simulink model "Hand_Made_PID"  (R2019a)
settings: Solver=VariableStepAuto  StartTime=0.0  StopTime=10.0  RelTol=1e-3
settings Model: Creator=hodam  LastModifiedBy=hodam

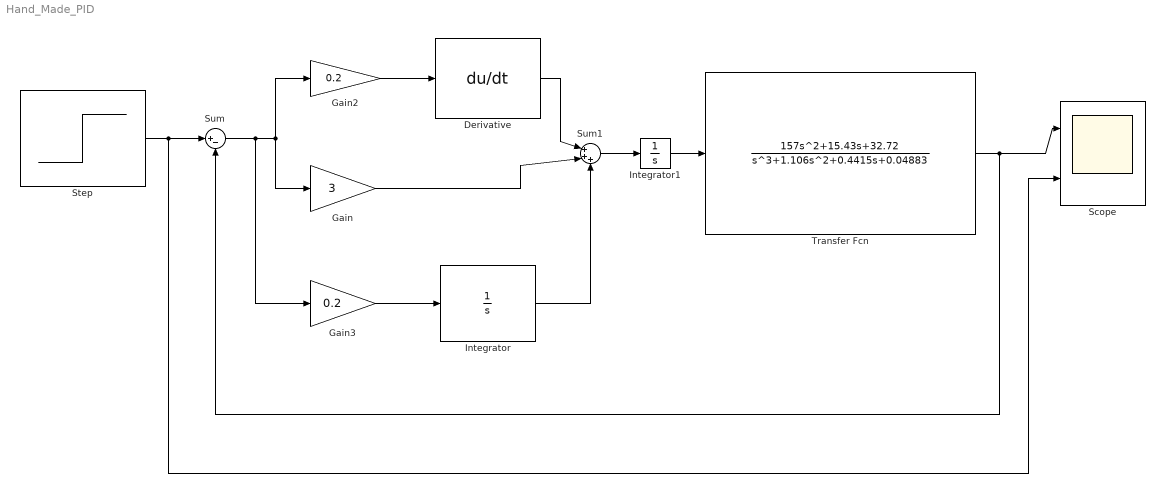
== system Hand_Made_PID ==
  Derivative : Derivative
  Gain : Gain  Gain=3
  Gain2 : Gain  Gain=0.2
  Gain3 : Gain  Gain=0.2
  Integrator : Integrator
  Integrator1 : Integrator
  Scope : Scope  NumInputPorts=2
  Step : Step  Time=0  After=60  SampleTime=0
  Sum : Sum  Inputs=|+-
  Sum1 : Sum  Inputs=|+++
  Transfer Fcn : TransferFcn  Numerator=[157 15.43 32.72]  Denominator=[1 1.106 0.4415 0.04883]
  wires:
  Derivative/1 -> Sum1/1
  Integrator/1 -> Sum1/3
  Gain/1 -> Sum1/2
  Gain3/1 -> Integrator/1
  Gain2/1 -> Derivative/1
  Sum/1 -> Gain3/1, Gain2/1, Gain/1
  Transfer Fcn/1 -> Sum/2, Scope/1
  Sum1/1 -> Integrator1/1
  Integrator1/1 -> Transfer Fcn/1
  Step/1 -> Scope/2, Sum/1
